simulink model "VIPRExit557StEnCtrl"  (R2018b)
settings: Solver=FixedStepDiscrete  StartTime=0.0  StopTime=10.0  FixedStep=0.01  RelTol=1e-3
undefined symbols (not defined in the file or in its folder): data, KeSMSw4SSecRwLtStLgrstOtwdInwdClosePos1_Val, KeSMSw4SSecRwLtStLgrstUpwdDnwdClosePos1_Val, KeSMSw4SSecRwLtStLgrstUpwdDnwdClosePos2_Val, KeSMSw4SSecRwLtStLgrstUpwdDnwdOpenPos1_Val, PassStBkReclnEn_Clear, PassStBkReclnEn_Set, PassStFwdBkwdEn_Clear, PassStFwdBkwdEn_Set, SecRwRtStBkReclnEn_Clear, SecRwRtStBkReclnEn_Set, SecRwRtStFwdBkwdEn_Clear, SecRwRtStFwdBkwdEn_Set, SecRwRtStLgrstInwdOtwdEn_Clear, SecRwRtStLgrstInwdOtwdEn_Set, SecRwRtStLgrstUpwdDnwdEn_Clear, SecRwRtStLgrstUpwdDnwdEn_Set, ThdRwLtStBkReclnEn_Clear, ThdRwLtStBkReclnEn_Set, ThdRwLtStFwdBkwdEn_Clear, ThdRwLtStFwdBkwdEn_Set, ThdRwRtStBkReclnEn_Clear, ThdRwRtStBkReclnEn_Set, ThdRwRtStFwdBkwdEn_Clear, ThdRwRtStFwdBkwdEn_Set, ZeroREn_Clear, ZeroREn_Set
libraries: simulink x1
settings Model: Creator=sn2xws  LastModifiedBy=sn2xws
settings Model: ModifiedHistory=|
  | 2024.7.4 V3.0.0 557模式流程V1.9
  | 2024.8.21 V3.0.1 增加FirstTrig参数
  | 2024.8.28 V3.0.2 副驾靠背小于目标位置时也要判断完成避免ongoing
  | 2024.9.18 V3.0.3  6s版本不需要动三左座椅，不需要posdone，第三阶段遗漏副驾靠背运动,三排占座不用动三排座椅，第三阶段遗漏三排靠背展开
  | 2024.9.18 V3.0.4 腿托及腿托延伸到位置信号连接错误
  | 2024.9.24 V3.0.5 7s版本三左靠背未到位置就到了下个阶段（进入第二阶段判断is7s改为！is7s），第三阶段未移动三左靠背
  | 2024.10.8 V3.0.6 方向比较常量类型错误
  | 25.9.12 V3.16.0 优化副驾占座逻辑，一旦占座不恢复动作
settings DataIOCC: SaveFormat=StructureWithTime
settings OptimizationCC: DefaultParameterBehavior=Inlined  EnhancedBackFolding=on  PassReuseOutputArgsAs=Individual arguments  ZeroExternalMemoryAtStartup=off  ZeroInternalMemoryAtStartup=off  OptimizeBlockOrder=speed  DifferentSizesBufferReuse=on  OptimizationCustomize=off
settings DebuggingCC: ParameterTunabilityLossMsg=error
settings SFSimCC: MATLABDynamicMemAlloc=off
settings RTWCC: SystemTargetFile=autosar.tlc  GenCodeOnly=on  TemplateMakefile=ert_default_tmf  Description=AUTOSAR  GenerateReport=on  IncludeHyperlinkInReport=on  LaunchReport=on  GenerateTraceInfo=on  GenerateTraceReport=on  GenerateTraceReportSl=on  GenerateTraceReportSf=on  GenerateTraceReportEml=on
settings CodeAppCC: ForceParamTrailComments=on  IgnoreCustomStorageClasses=off  OperatorAnnotations=on  SimulinkDataObjDesc=on  SFDataObjDesc=on  InsertBlockDesc=on
settings STFCustomTargetCC: TargetLangStandard=C99 (ISO)  MultiwordLength=256  ParMdlRefBuildCompliant=on  CompOptLevelCompliant=on  IncludeMdlTerminateFcn=off  CombineOutputUpdateFcns=on  SuppressErrorStatus=on  ERTCustomFileBanners=on  SupportNonFinite=off  SupportComplex=off  SupportContinuousTime=off  SupportNonInlinedSFcns=off  RemoveResetFunc=on  MATLABClassNameForMDSCustomization=Simulink.SoftwareTarget.ERTCustomization  AutosarCompliant=on  UseToolchainInfoCompliant=on  LookupTableObjectStructAxisOrder=2,1,3,4,...  LUTObjectStructOrderEvenSpacing=Size,Table,Breakpoints  SystemTargetFile=autosar.tlc
settings ERTTargetCC: TargetLangStandard=C99 (ISO)  ConcurrentExecutionCompliant=off  IncludeMdlTerminateFcn=off  SuppressErrorStatus=on  SupportNonFinite=off  SupportComplex=off  ModelStepFunctionPrototypeControlCompliant=off  CPPClassGenCompliant=off  AutosarCompliant=on  LookupTableObjectStructAxisOrder=2,1,3,4,...  LUTObjectStructOrderEvenSpacing=Size,Table,Breakpoints  InlinedParameterPlacement=NonHierarchical  ERTCustomFileTemplate=example_file_process.tlc  ERTFilePackagingFormat=Compact

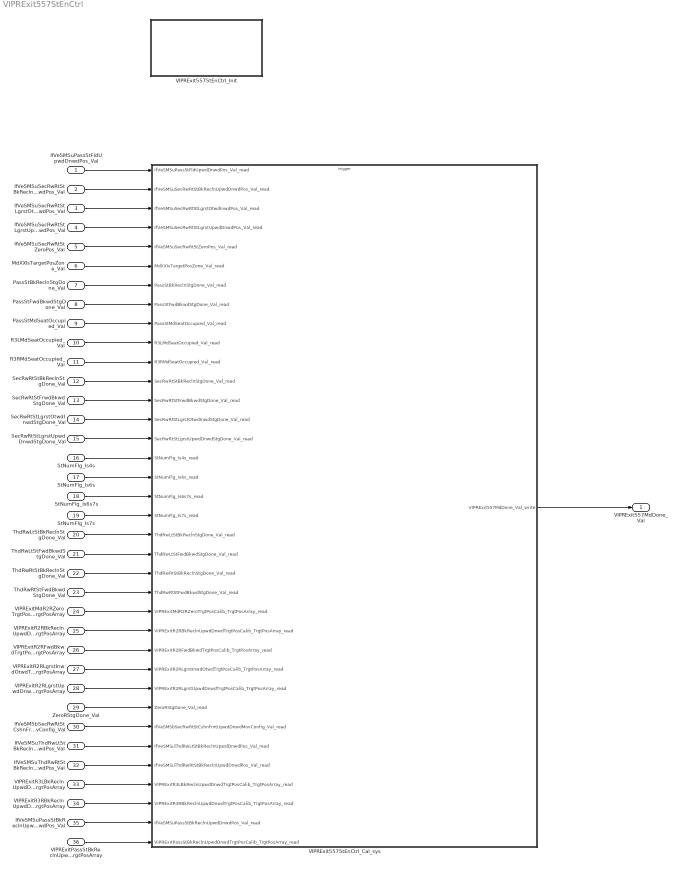
== system VIPRExit557StEnCtrl ==
  IfVeSMSuPassStFldUpwdDnwdPos_Val : Inport  OutDataTypeStr=uint16  PortDimensions=1
  IfVeSMSuSecRwRtStBkReclnUpwdDnwdPos_Val : Inport  Port=2  OutDataTypeStr=uint16  PortDimensions=1
  IfVeSMSuSecRwRtStLgrstOtwdInwdPos_Val : Inport  Port=3  OutDataTypeStr=uint16  PortDimensions=1
  IfVeSMSuSecRwRtStLgrstUpwdDnwdPos_Val : Inport  Port=4  OutDataTypeStr=uint16  PortDimensions=1
  IfVeSMSuSecRwRtStZeroPos_Val : Inport  Port=5  OutDataTypeStr=uint16  PortDimensions=1
  MdXXIsTargetPosZone_Val : Inport  Port=6  OutDataTypeStr=uint32  PortDimensions=1
  PassStBkReclnStgDone_Val : Inport  Port=7  OutDataTypeStr=boolean  PortDimensions=1
  PassStFwdBkwdStgDone_Val : Inport  Port=8  OutDataTypeStr=boolean  PortDimensions=1
  PassStMdSeatOccupied_Val : Inport  Port=9  OutDataTypeStr=boolean  PortDimensions=1
  R3LMdSeatOccupied_Val : Inport  Port=10  OutDataTypeStr=boolean  PortDimensions=1
  R3RMdSeatOccupied_Val : Inport  Port=11  OutDataTypeStr=boolean  PortDimensions=1
  SecRwRtStBkReclnStgDone_Val : Inport  Port=12  OutDataTypeStr=boolean  PortDimensions=1
  SecRwRtStFrwdBkwdStgDone_Val : Inport  Port=13  OutDataTypeStr=boolean  PortDimensions=1
  SecRwRtStLgrstOtwdInwdStgDone_Val : Inport  Port=14  OutDataTypeStr=boolean  PortDimensions=1
  SecRwRtStLgrstUpwdDnwdStgDone_Val : Inport  Port=15  OutDataTypeStr=boolean  PortDimensions=1
  StNumFlg_Is4s : Inport  Port=16  OutDataTypeStr=boolean  PortDimensions=1
  StNumFlg_Is6s : Inport  Port=17  OutDataTypeStr=boolean  PortDimensions=1
  StNumFlg_Is6s7s : Inport  Port=18  OutDataTypeStr=boolean  PortDimensions=1
  StNumFlg_Is7s : Inport  Port=19  OutDataTypeStr=boolean  PortDimensions=1
  ThdRwLtStBkReclnStgDone_Val : Inport  Port=20  OutDataTypeStr=boolean  PortDimensions=1
  ThdRwLtStFwdBkwdStgDone_Val : Inport  Port=21  OutDataTypeStr=boolean  PortDimensions=1
  ThdRwRtStBkReclnStgDone_Val : Inport  Port=22  OutDataTypeStr=boolean  PortDimensions=1
  ThdRwRtStFwdBkwdStgDone_Val : Inport  Port=23  OutDataTypeStr=boolean  PortDimensions=1
  VIPRExitMdR2RZeroTrgtPosCalib_TrgtPosArray : Inport  Description=|  Port=24  OutDataTypeStr=uint16  PortDimensions=3
      | 0:Pos
      | 1:Max
      | 2:Min
  VIPRExitR2RBkReclnUpwdDnwdTrgtPosCalib_TrgtPosArray : Inport  Description=|  Port=25  OutDataTypeStr=uint16  PortDimensions=3
      | 0:Pos
      | 1:Max
      | 2:Min
  VIPRExitR2RFwdBkwdTrgtPosCalib_TrgtPosArray : Inport  Description=|  Port=26  OutDataTypeStr=uint16  PortDimensions=3
      | 0:Pos
      | 1:Max
      | 2:Min
  VIPRExitR2RLgrstInwdOtwdTrgtPosCalib_TrgtPosArray : Inport  Description=|  Port=27  OutDataTypeStr=uint16  PortDimensions=3
      | 0:Pos
      | 1:Max
      | 2:Min
  VIPRExitR2RLgrstUpwdDnwdTrgtPosCalib_TrgtPosArray : Inport  Description=|  Port=28  OutDataTypeStr=uint16  PortDimensions=3
      | 0:Pos
      | 1:Max
      | 2:Min
  ZeroRStgDone_Val : Inport  Port=29  OutDataTypeStr=boolean  PortDimensions=1
  IfVeSMSbSecRwRtStCshnFrntUpwdDnwdMovConfig_Val : Inport  Port=30  OutDataTypeStr=boolean  PortDimensions=1
  IfVeSMSuThdRwLtStBkReclnUpwdDnwdPos_Val : Inport  Port=31  OutDataTypeStr=uint16  PortDimensions=1
  IfVeSMSuThdRwRtStBkReclnUpwdDnwdPos_Val : Inport  Port=32  OutDataTypeStr=uint16  PortDimensions=1
  VIPRExitR3LBkReclnUpwdDnwdTrgtPosCalib_TrgtPosArray : Inport  Description=|  Port=33  OutDataTypeStr=uint16  PortDimensions=3
      | 0:Pos
      | 1:Max
      | 2:Min
  VIPRExitR3RBkReclnUpwdDnwdTrgtPosCalib_TrgtPosArray : Inport  Description=|  Port=34  OutDataTypeStr=uint16  PortDimensions=3
      | 0:Pos
      | 1:Max
      | 2:Min
  IfVeSMSuPassStBkReclnUpwdDnwdPos_Val : Inport  Port=35  OutDataTypeStr=uint16  PortDimensions=1
  VIPRExitPassStBkReclnUpwdDnwdTrgtPosCalib_TrgtPosArray : Inport  Description=|  Port=36  OutDataTypeStr=uint16  PortDimensions=3
      | 0:Pos
      | 1:Max
      | 2:Min
  VIPRExit557StEnCtrl_Cal_sys : Subsystem
  VIPRExit557StEnCtrl_Init : Subsystem
  VIPRExit557MdDone_Val : Outport  OutDataTypeStr=uint8  PortDimensions=1
  wires:
  IfVeSMSuPassStFldUpwdDnwdPos_Val/1 -> VIPRExit557StEnCtrl_Cal_sys/1(IfVeSMSuPassStFldUpwdDnwdPos_Val_read)
  IfVeSMSuSecRwRtStBkReclnUpwdDnwdPos_Val/1 -> VIPRExit557StEnCtrl_Cal_sys/2(IfVeSMSuSecRwRtStBkReclnUpwdDnwdPos_Val_read)
  IfVeSMSuSecRwRtStLgrstOtwdInwdPos_Val/1 -> VIPRExit557StEnCtrl_Cal_sys/3(IfVeSMSuSecRwRtStLgrstOtwdInwdPos_Val_read)
  IfVeSMSuSecRwRtStLgrstUpwdDnwdPos_Val/1 -> VIPRExit557StEnCtrl_Cal_sys/4(IfVeSMSuSecRwRtStLgrstUpwdDnwdPos_Val_read)
  IfVeSMSuSecRwRtStZeroPos_Val/1 -> VIPRExit557StEnCtrl_Cal_sys/5(IfVeSMSuSecRwRtStZeroPos_Val_read)
  MdXXIsTargetPosZone_Val/1 -> VIPRExit557StEnCtrl_Cal_sys/6(MdXXIsTargetPosZone_Val_read)
  PassStBkReclnStgDone_Val/1 -> VIPRExit557StEnCtrl_Cal_sys/7(PassStBkReclnStgDone_Val_read)
  PassStFwdBkwdStgDone_Val/1 -> VIPRExit557StEnCtrl_Cal_sys/8(PassStFwdBkwdStgDone_Val_read)
  PassStMdSeatOccupied_Val/1 -> VIPRExit557StEnCtrl_Cal_sys/9(PassStMdSeatOccupied_Val_read)
  R3LMdSeatOccupied_Val/1 -> VIPRExit557StEnCtrl_Cal_sys/10(R3LMdSeatOccupied_Val_read)
  R3RMdSeatOccupied_Val/1 -> VIPRExit557StEnCtrl_Cal_sys/11(R3RMdSeatOccupied_Val_read)
  SecRwRtStBkReclnStgDone_Val/1 -> VIPRExit557StEnCtrl_Cal_sys/12(SecRwRtStBkReclnStgDone_Val_read)
  SecRwRtStFrwdBkwdStgDone_Val/1 -> VIPRExit557StEnCtrl_Cal_sys/13(SecRwRtStFrwdBkwdStgDone_Val_read)
  SecRwRtStLgrstOtwdInwdStgDone_Val/1 -> VIPRExit557StEnCtrl_Cal_sys/14(SecRwRtStLgrstOtwdInwdStgDone_Val_read)
  SecRwRtStLgrstUpwdDnwdStgDone_Val/1 -> VIPRExit557StEnCtrl_Cal_sys/15(SecRwRtStLgrstUpwdDnwdStgDone_Val_read)
  StNumFlg_Is4s/1 -> VIPRExit557StEnCtrl_Cal_sys/16(StNumFlg_Is4s_read)
  StNumFlg_Is6s/1 -> VIPRExit557StEnCtrl_Cal_sys/17(StNumFlg_Is6s_read)
  StNumFlg_Is6s7s/1 -> VIPRExit557StEnCtrl_Cal_sys/18(StNumFlg_Is6s7s_read)
  StNumFlg_Is7s/1 -> VIPRExit557StEnCtrl_Cal_sys/19(StNumFlg_Is7s_read)
  ThdRwLtStBkReclnStgDone_Val/1 -> VIPRExit557StEnCtrl_Cal_sys/20(ThdRwLtStBkReclnStgDone_Val_read)
  ThdRwLtStFwdBkwdStgDone_Val/1 -> VIPRExit557StEnCtrl_Cal_sys/21(ThdRwLtStFwdBkwdStgDone_Val_read)
  ThdRwRtStBkReclnStgDone_Val/1 -> VIPRExit557StEnCtrl_Cal_sys/22(ThdRwRtStBkReclnStgDone_Val_read)
  ThdRwRtStFwdBkwdStgDone_Val/1 -> VIPRExit557StEnCtrl_Cal_sys/23(ThdRwRtStFwdBkwdStgDone_Val_read)
  VIPRExitMdR2RZeroTrgtPosCalib_TrgtPosArray/1 -> VIPRExit557StEnCtrl_Cal_sys/24(VIPRExitMdR2RZeroTrgtPosCalib_TrgtPosArray_read)
  VIPRExitR2RBkReclnUpwdDnwdTrgtPosCalib_TrgtPosArray/1 -> VIPRExit557StEnCtrl_Cal_sys/25(VIPRExitR2RBkReclnUpwdDnwdTrgtPosCalib_TrgtPosArray_read)
  VIPRExitR2RFwdBkwdTrgtPosCalib_TrgtPosArray/1 -> VIPRExit557StEnCtrl_Cal_sys/26(VIPRExitR2RFwdBkwdTrgtPosCalib_TrgtPosArray_read)
  VIPRExitR2RLgrstInwdOtwdTrgtPosCalib_TrgtPosArray/1 -> VIPRExit557StEnCtrl_Cal_sys/27(VIPRExitR2RLgrstInwdOtwdTrgtPosCalib_TrgtPosArray_read)
  VIPRExitR2RLgrstUpwdDnwdTrgtPosCalib_TrgtPosArray/1 -> VIPRExit557StEnCtrl_Cal_sys/28(VIPRExitR2RLgrstUpwdDnwdTrgtPosCalib_TrgtPosArray_read)
  ZeroRStgDone_Val/1 -> VIPRExit557StEnCtrl_Cal_sys/29(ZeroRStgDone_Val_read)
  VIPRExit557StEnCtrl_Cal_sys/1(VIPRExit557MdDone_Val_write) -> VIPRExit557MdDone_Val/1
  IfVeSMSbSecRwRtStCshnFrntUpwdDnwdMovConfig_Val/1 -> VIPRExit557StEnCtrl_Cal_sys/30(IfVeSMSbSecRwRtStCshnFrntUpwdDnwdMovConfig_Val_read)
  IfVeSMSuThdRwLtStBkReclnUpwdDnwdPos_Val/1 -> VIPRExit557StEnCtrl_Cal_sys/31(IfVeSMSuThdRwLtStBkReclnUpwdDnwdPos_Val_read)
  IfVeSMSuThdRwRtStBkReclnUpwdDnwdPos_Val/1 -> VIPRExit557StEnCtrl_Cal_sys/32(IfVeSMSuThdRwRtStBkReclnUpwdDnwdPos_Val_read)
  VIPRExitR3LBkReclnUpwdDnwdTrgtPosCalib_TrgtPosArray/1 -> VIPRExit557StEnCtrl_Cal_sys/33(VIPRExitR3LBkReclnUpwdDnwdTrgtPosCalib_TrgtPosArray_read)
  VIPRExitR3RBkReclnUpwdDnwdTrgtPosCalib_TrgtPosArray/1 -> VIPRExit557StEnCtrl_Cal_sys/34(VIPRExitR3RBkReclnUpwdDnwdTrgtPosCalib_TrgtPosArray_read)
  IfVeSMSuPassStBkReclnUpwdDnwdPos_Val/1 -> VIPRExit557StEnCtrl_Cal_sys/35(IfVeSMSuPassStBkReclnUpwdDnwdPos_Val_read)
  VIPRExitPassStBkReclnUpwdDnwdTrgtPosCalib_TrgtPosArray/1 -> VIPRExit557StEnCtrl_Cal_sys/36(VIPRExitPassStBkReclnUpwdDnwdTrgtPosCalib_TrgtPosArray_read)

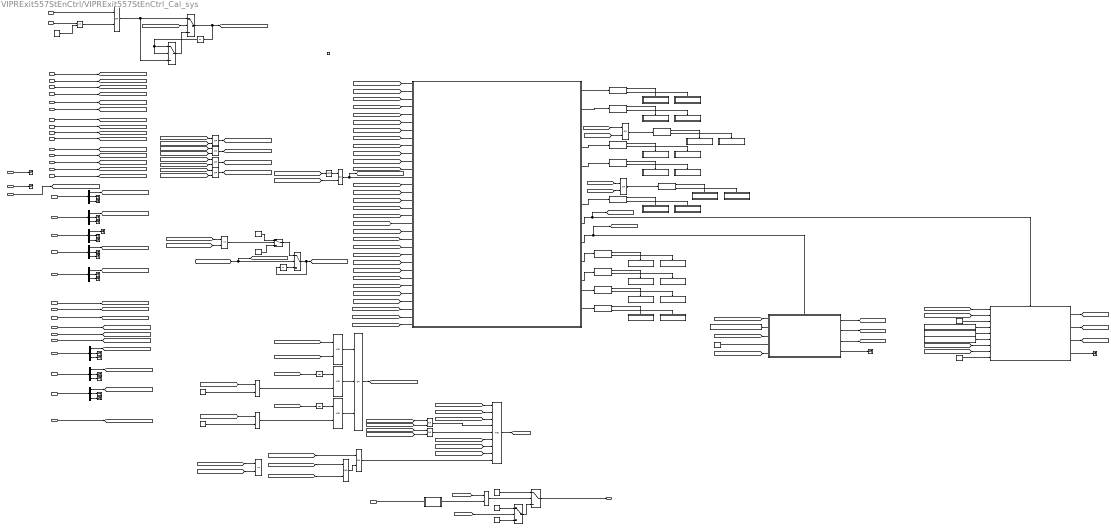
== system VIPRExit557StEnCtrl/VIPRExit557StEnCtrl_Cal_sys ==
  IfVeSMSuPassStFldUpwdDnwdPos_Val_read : Inport
  IfVeSMSuSecRwRtStBkReclnUpwdDnwdPos_Val_read : Inport  Port=2
  IfVeSMSuSecRwRtStLgrstOtwdInwdPos_Val_read : Inport  Port=3
  IfVeSMSuSecRwRtStLgrstUpwdDnwdPos_Val_read : Inport  Port=4
  IfVeSMSuSecRwRtStZeroPos_Val_read : Inport  Port=5
  MdXXIsTargetPosZone_Val_read : Inport  Port=6
  PassStBkReclnStgDone_Val_read : Inport  Port=7
  PassStFwdBkwdStgDone_Val_read : Inport  Port=8
  PassStMdSeatOccupied_Val_read : Inport  Port=9
  R3LMdSeatOccupied_Val_read : Inport  Port=10
  R3RMdSeatOccupied_Val_read : Inport  Port=11
  SecRwRtStBkReclnStgDone_Val_read : Inport  Port=12
  SecRwRtStFrwdBkwdStgDone_Val_read : Inport  Port=13
  SecRwRtStLgrstOtwdInwdStgDone_Val_read : Inport  Port=14
  SecRwRtStLgrstUpwdDnwdStgDone_Val_read : Inport  Port=15
  StNumFlg_Is4s_read : Inport  Port=16
  StNumFlg_Is6s_read : Inport  Port=17
  StNumFlg_Is6s7s_read : Inport  Port=18
  StNumFlg_Is7s_read : Inport  Port=19
  ThdRwLtStBkReclnStgDone_Val_read : Inport  Port=20
  ThdRwLtStFwdBkwdStgDone_Val_read : Inport  Port=21
  ThdRwRtStBkReclnStgDone_Val_read : Inport  Port=22
  ThdRwRtStFwdBkwdStgDone_Val_read : Inport  Port=23
  VIPRExitMdR2RZeroTrgtPosCalib_TrgtPosArray_read : Inport  Port=24
  VIPRExitR2RBkReclnUpwdDnwdTrgtPosCalib_TrgtPosArray_read : Inport  Port=25
  VIPRExitR2RFwdBkwdTrgtPosCalib_TrgtPosArray_read : Inport  Port=26
  VIPRExitR2RLgrstInwdOtwdTrgtPosCalib_TrgtPosArray_read : Inport  Port=27
  VIPRExitR2RLgrstUpwdDnwdTrgtPosCalib_TrgtPosArray_read : Inport  Port=28
  ZeroRStgDone_Val_read : Inport  Port=29
  IfVeSMSbSecRwRtStCshnFrntUpwdDnwdMovConfig_Val_read : Inport  Port=30
  IfVeSMSuThdRwLtStBkReclnUpwdDnwdPos_Val_read : Inport  Port=31
  IfVeSMSuThdRwRtStBkReclnUpwdDnwdPos_Val_read : Inport  Port=32
  VIPRExitR3LBkReclnUpwdDnwdTrgtPosCalib_TrgtPosArray_read : Inport  Port=33
  VIPRExitR3RBkReclnUpwdDnwdTrgtPosCalib_TrgtPosArray_read : Inport  Port=34
  IfVeSMSuPassStBkReclnUpwdDnwdPos_Val_read : Inport  Port=35
  VIPRExitPassStBkReclnUpwdDnwdTrgtPosCalib_TrgtPosArray_read : Inport  Port=36
  function : TriggerPort  TriggerType=function-call  IsSimulinkFunction=on  FunctionName=VIPRExit557StEnCtrl_Cal  VariantControl=(inherit)
  32BitSelector : Subsystem  mask(32 Bit Selector){BitNum=27}
      mask prompts: BitNum "Select Bit Number"
      mask help: Allows selection of a particular bit (0-31) out of a packed word up to 32 bits long. Output will be true if the bit number selected via the mask parameter is equal to one.
      mask TypeOptions BitNum: 0 | 1 | 2 | 3 | 4 | 5 | 6 | 7 | 8 | 9 | 10 | 11 | 12 | 13 | 14 | 15 | 16 | 17 | 18 | 19 | 20 | 21 | 22 | 23 | 24 | 25 | 26 | 27 | 28 | 29 | 30 | 31
      mask Display:
      | text(0.5, 0.8,'BIT','horizontalAlignment','center')
      | text(0.5, 0.5,'SELECTOR','horizontalAlignment','center')
      | text(0.5, 0.2,['-- Bit ',char(get_param(gcb,'BitNum')),' --'],'horizontalAlignment','center')
  Chart : Stateflow chart  TreatAsAtomicUnit=on
  Constant : Constant  OutDataTypeStr=uint8
  Constant1 : Constant  Value=2  OutDataTypeStr=uint8
  Constant10 : Constant  OutDataTypeStr=uint8
  Constant11 : Constant  Value=0  OutDataTypeStr=uint16
  Constant2 : Constant  Value=0  OutDataTypeStr=uint8
  Constant3 : Constant  OutDataTypeStr=boolean
  Constant4 : Constant  OutDataTypeStr=boolean
  Constant5 : Constant  Value=0  OutDataTypeStr=uint16
  Constant7 : Constant  OutDataTypeStr=uint8
  Constant8 : Constant  Value=2  OutDataTypeStr=uint8
  Constant9 : Constant  Value=2  OutDataTypeStr=uint8
  Demux{,1..7} (8 alike) : Demux  Outputs=3
  If Action Subsystem1 : Subsystem  TreatAsAtomicUnit=on
  If Action Subsystem10 : Subsystem  TreatAsAtomicUnit=on
  If Action Subsystem11 : Subsystem  TreatAsAtomicUnit=on
  If Action Subsystem12 : Subsystem  TreatAsAtomicUnit=on
  If Action Subsystem13 : Subsystem  TreatAsAtomicUnit=on
  If Action Subsystem14 : Subsystem  TreatAsAtomicUnit=on
  If Action Subsystem15 : Subsystem  TreatAsAtomicUnit=on
  If Action Subsystem16 : Subsystem  TreatAsAtomicUnit=on
  If Action Subsystem17 : Subsystem  TreatAsAtomicUnit=on
  If Action Subsystem18 : Subsystem  TreatAsAtomicUnit=on
  If Action Subsystem19 : Subsystem  TreatAsAtomicUnit=on
  If Action Subsystem2 : Subsystem  TreatAsAtomicUnit=on
  If Action Subsystem20 : Subsystem  TreatAsAtomicUnit=on
  If Action Subsystem21 : Subsystem  TreatAsAtomicUnit=on
  If Action Subsystem22 : Subsystem  TreatAsAtomicUnit=on
  If Action Subsystem3 : Subsystem  TreatAsAtomicUnit=on
  If Action Subsystem4 : Subsystem  TreatAsAtomicUnit=on
  If Action Subsystem5 : Subsystem  TreatAsAtomicUnit=on
  If Action Subsystem6 : Subsystem  TreatAsAtomicUnit=on
  If Action Subsystem7 : Subsystem  TreatAsAtomicUnit=on
  If Action Subsystem8 : Subsystem  TreatAsAtomicUnit=on
  If Action Subsystem9 : Subsystem  TreatAsAtomicUnit=on
  If{1..11} (11 alike) : If  IfExpression=u1
  LgrstClose : Subsystem
  LgrstOpen : Subsystem
  Logical Operator : Logic  Operator=NOT  AllPortsSameDT=off  OutDataTypeStr=boolean
  Logical Operator{1,3..4,12..19} (11 alike) : Logic  Operator=OR  AllPortsSameDT=off  OutDataTypeStr=boolean
  Logical Operator10 : Logic  Inputs=9  AllPortsSameDT=off  OutDataTypeStr=boolean
  Logical Operator{2,6..7,9,11} (5 alike) : Logic  AllPortsSameDT=off  OutDataTypeStr=boolean
  Logical Operator5 : Logic  Operator=OR  Inputs=3  AllPortsSameDT=off  OutDataTypeStr=boolean
  PA_KeSMSw4SSecRwLtStLgrstOtwdInwdClosePos1_Val : Constant  Value=KeSMSw4SSecRwLtStLgrstOtwdInwdClosePos1_Val
  PA_KeSMSw4SSecRwLtStLgrstUpwdDnwdClosePos1_Val : Constant  Value=KeSMSw4SSecRwLtStLgrstUpwdDnwdClosePos1_Val
  PA_KeSMSw4SSecRwLtStLgrstUpwdDnwdClosePos2_Val : Constant  Value=KeSMSw4SSecRwLtStLgrstUpwdDnwdClosePos2_Val
  PA_KeSMSw4SSecRwLtStLgrstUpwdDnwdOpenPos1_Val1 : Constant  Value=KeSMSw4SSecRwLtStLgrstUpwdDnwdOpenPos1_Val
  Relational Operator : RelationalOperator  OutDataTypeStr=boolean  RndMeth=Simplest
  Relational Operator1 : RelationalOperator  Operator===  OutDataTypeStr=boolean  RndMeth=Simplest
  Relational Operator2 : RelationalOperator  Operator=<=  OutDataTypeStr=boolean  RndMeth=Simplest
  Relational Operator3 : RelationalOperator  Operator===  OutDataTypeStr=boolean  RndMeth=Simplest
  Relational Operator4 : RelationalOperator  Operator=<=  OutDataTypeStr=boolean  RndMeth=Simplest
  Switch{,1..5} (6 alike) : Switch  Criteria=u2 > Threshold
  Terminator{,1..10,12..21} (21 alike) : Terminator
  Unit Delay{,1,3..4} (4 alike) : UnitDelay  SampleTime=-1
  FirstTrig : ArgIn  OutDataTypeStr=boolean  ArgumentName=FirstTrig
  VIPRExit557MdDone_Val_write : Outport
      settings: EnsureOutportIsVirtual=on
  wires:
  Switch/1 -> VIPRExit557MdDone_Val_write/1
  ZeroRStgDone_Val_read/1 -> [ZeroRStgDone]
  PassStFwdBkwdStgDone_Val_read/1 -> [PassStFwdBkwdStgDone]
  IfVeSMSuSecRwRtStZeroPos_Val_read/1 -> [IfVeSMSuSecRwRtStZeroPos]
  SecRwRtStFrwdBkwdStgDone_Val_read/1 -> [SecRwRtStFrwdBkwdStgDone]
  ThdRwLtStBkReclnStgDone_Val_read/1 -> [ThdRwLtStBkReclnStgDone]
  IfVeSMSuSecRwRtStLgrstUpwdDnwdPos_Val_read/1 -> [IfVeSMSuSecRwRtStLgrstUpwdDnwdPos]
  IfVeSMSuSecRwRtStLgrstOtwdInwdPos_Val_read/1 -> [IfVeSMSuSecRwRtStLgrstOtwdInwdPos]
  ThdRwLtStFwdBkwdStgDone_Val_read/1 -> [ThdRwLtStFwdBkwdStgDone]
  SecRwRtStBkReclnStgDone_Val_read/1 -> [SecRwRtStBkReclnStgDone]
  IfVeSMSuSecRwRtStBkReclnUpwdDnwdPos_Val_read/1 -> [IfVeSMSuSecRwRtStBkReclnUpwdDnwdPos]
  PassStBkReclnStgDone_Val_read/1 -> [PassStBkReclnStgDone]
  ThdRwRtStBkReclnStgDone_Val_read/1 -> [ThdRwRtStBkReclnStgDone]
  ThdRwRtStFwdBkwdStgDone_Val_read/1 -> [ThdRwRtStFwdBkwdStgDone]
  VIPRExitR2RFwdBkwdTrgtPosCalib_TrgtPosArray_read/1 -> Demux1/1
  Demux1/3 -> Terminator3/1
  Demux/2 -> Terminator/1
  Demux3/2 -> Terminator6/1
  Demux2/2 -> Terminator4/1
  Demux1/1 -> Terminator15/1
  Demux4/2 -> Terminator8/1
  Demux/3 -> Terminator1/1
  VIPRExitMdR2RZeroTrgtPosCalib_TrgtPosArray_read/1 -> Demux4/1
  VIPRExitR2RLgrstUpwdDnwdTrgtPosCalib_TrgtPosArray_read/1 -> Demux3/1
  Demux3/1 -> [VIPRR2RLgrstUpwdDnwdTrgtPos]
  Demux1/2 -> Terminator2/1
  Demux2/1 -> [VIPRR2RLgrstInwdOtwdTrgtPos]
  Demux3/3 -> Terminator7/1
  VIPRExitR2RLgrstInwdOtwdTrgtPosCalib_TrgtPosArray_read/1 -> Demux2/1
  Demux2/3 -> Terminator5/1
  Demux/1 -> [VIPRR2RBkReclnUpwdDnwdTrgtPos]
  Demux4/1 -> [VIPRMdR2RZeroTrgtPos]
  VIPRExitR2RBkReclnUpwdDnwdTrgtPosCalib_TrgtPosArray_read/1 -> Demux/1
  Demux4/3 -> Terminator9/1
  StNumFlg_Is4s_read/1 -> Terminator10/1
  StNumFlg_Is6s_read/1 -> [is6s]
  StNumFlg_Is6s7s_read/1 -> Terminator12/1
  R3LMdSeatOccupied_Val_read/1 -> [R3LMdSeatOccupied]
  R3RMdSeatOccupied_Val_read/1 -> [R3RMdSeatOccupied]
  StNumFlg_Is7s_read/1 -> [StNumFlg_Is7s]
  MdXXIsTargetPosZone_Val_read/1 -> 32BitSelector/1(x)
  [AllDone] -> Logical Operator9/1
  Constant1/1 -> Switch1/1
  [AllDone] -> Switch1/2
  Switch1/1 -> Switch/3
  Constant/1 -> Switch/1
  Logical Operator9/1 -> Switch/2
  32BitSelector/1(y) -> Logical Operator9/2
  Constant2/1 -> Switch1/3
  PA_KeSMSw4SSecRwLtStLgrstUpwdDnwdOpenPos1_Val1/1 -> LgrstOpen/2(LgrstUpwdDnwdOpenPos1)
  PA_KeSMSw4SSecRwLtStLgrstUpwdDnwdClosePos2_Val/1 -> LgrstClose/5(LgrstUpwdDnwdClosePos2)
  Constant5/1 -> LgrstClose/3(FtupwdDnwdPos)
  Constant4/1 -> LgrstClose/9(FtrstStgDone)
  [IfVeSMSuSecRwRtStLgrstOtwdInwdPos] -> LgrstClose/2(LgrstInwdOtwdPos)
  Logical Operator3/1 -> If4/1
  Chart/9(LgrstOpnEn) -> [LgrstOpnEn], LgrstOpen/Enable
  If1/2 -> If Action Subsystem1/Action
  Chart/5(ThdRwLtStFwdBkwdEn) -> If3/1
  LgrstOpen/4(FtrstEn) -> Terminator14/1
  PA_KeSMSw4SSecRwLtStLgrstOtwdInwdClosePos1_Val/1 -> LgrstClose/6(LgrstInwdOtWdPos1)
  Chart/8(LgrstClsEn) -> LgrstClose/Enable, [LgrstClsEn]
  [LgrstUpwdEn3] -> Logical Operator3/2
  Chart/2(SecRwLtStFrwdBkwdEn) -> If1/1
  Logical Operator4/1 -> If5/1
  Chart/1(SecRwLtStBkReclnEn) -> If8/1
  LgrstOpen/1(Failflg) -> [FailflgOpn]
  If1/1 -> If Action Subsystem2/Action
  If5/1 -> If Action Subsystem10/Action
  [LgrstInwdOtwdEn3] -> Logical Operator4/2
  If3/2 -> If Action Subsystem5/Action
  LgrstOpen/2(LgrstInwdOtwdEn) -> [LgrstInwdOtwdEn2]
  [IfVeSMSuSecRwRtStLgrstUpwdDnwdPos] -> LgrstClose/1(LgrstUpwdDnwdPos)
  If6/1 -> If Action Subsystem13/Action
  [LgrstInwdOtwdEn2] -> Logical Operator4/1
  If8/1 -> If Action Subsystem14/Action
  Constant3/1 -> LgrstOpen/4(FtrstStgDone)
  Chart/4(ThdRwLtStBkReclnEn) -> If2/1
  If2/1 -> If Action Subsystem4/Action
  If4/1 -> If Action Subsystem8/Action
  If8/2 -> If Action Subsystem11/Action
  [SecRwRtStLgrstUpwdDnwdStgDone] -> LgrstOpen/3(LgrstUpwdStgDone)
  PA_KeSMSw4SSecRwLtStLgrstUpwdDnwdClosePos1_Val/1 -> LgrstClose/4(LgrstUpwdDnwdClosePos1)
  If2/2 -> If Action Subsystem3/Action
  If5/2 -> If Action Subsystem9/Action
  If4/2 -> If Action Subsystem7/Action
  [LgrstUpwdEn2] -> Logical Operator3/1
  [SecRwRtStLgrstOtwdInwdStgDone] -> LgrstOpen/5(LgrstInwdStgDone)
  LgrstClose/2(LgrstInwdOtwdEn) -> [LgrstInwdOtwdEn3]
  If3/1 -> If Action Subsystem6/Action
  LgrstClose/4(FtrstEn) -> Terminator13/1
  [IfVeSMSuSecRwRtStLgrstUpwdDnwdPos] -> LgrstOpen/1(LgrstUpwdDnwdPos)
  LgrstOpen/3(LgrstUpwdDnwdEn) -> [LgrstUpwdEn2]
  Chart/7(ZeroLEn) -> If6/1
  [SecRwRtStLgrstUpwdDnwdStgDone] -> LgrstClose/8(LgrstUpwdStgDone)
  LgrstClose/3(LgrstUpwdDnwdEn) -> [LgrstUpwdEn3]
  [SecRwRtStLgrstOtwdInwdStgDone] -> LgrstClose/7(LgrstInwdStgDone)
  LgrstClose/1(Failflg) -> [FailflgCls]
  If6/2 -> If Action Subsystem12/Action
  [LgrstMoveDirection] -> Chart/19(LgrstMoveDirection)
  [SecRwRtStFrwdBkwdStgDone] -> Chart/5(SecRwLtStFrwdBkwdStgDone)
  [ThdRwLtStFwdBkwdStgDoneModify] -> Chart/9(ThdRwLtStFwdBkwdStgDone)
  [IfVeSMSuSecRwRtStLgrstOtwdInwdPos] -> Chart/2(IfVeSMSuSecRwLtStLgrstOtwdInwdPos)
  [IfVeSMSuThdRwLtStBkReclnUpwdDnwdPos] -> Chart/18(IfVeSMSuThdRwLtStBkReclnUpwdDnwdPos)
  [IfVeSMSuSecRwRtStLgrstUpwdDnwdPos] -> Relational Operator/1
  Relational Operator/1 -> Switch2/2
  [LgrstStgDone] -> Chart/17(LgrstStgDone)
  [VIPRR2RLgrstUpwdDnwdTrgtPos] -> Relational Operator/2
  [IfVeSMSuSecRwRtStZeroPos] -> Chart/14(IfVeSMSuSecRwLtStZeroPos)
  [R3LMdSeatOccupied] -> Chart/16(R3LMdSeatOccupied)
  [IfVeSMSbSecRwRtStCshnFrntUpwdDnwdMovConfig] -> Logical Operator/1
  [ZeroRStgDone] -> Logical Operator1/2
  Constant8/1 -> Switch2/3
  [VIPRR2RLgrstInwdOtwdTrgtPos] -> Chart/11(VIPLR2LLgrstInwdOtwdTrgtPos)
  [ThdRwLtStBkReclnStgDoneModify] -> Chart/8(ThdRwLtStBkReclnStgDone)
  [VIPRR2RLgrstUpwdDnwdTrgtPos] -> Chart/12(VIPLR2LLgrstUpwdDnwdTrgtPos)
  [SecRwRtStLgrstUpwdDnwdStgDone] -> Chart/7(SecRwLtStLgrstUpwdDnwdStgDone)
  [IfVeSMSuSecRwRtStBkReclnUpwdDnwdPos] -> Chart/1(IfVeSMSuSecRwLtStBkReclnUpwdDnwdPos)
  Constant7/1 -> Switch2/1
  Logical Operator1/1 -> [ZeroRStgDoneModify], Chart/13(ZeroLStgDone)
  [SecRwRtStBkReclnStgDone] -> Chart/4(SecRwLtStBkReclnStgDone)
  Logical Operator/1 -> Logical Operator1/1
  [SecRwRtStLgrstOtwdInwdStgDone] -> Chart/6(SecRwLtStLgrstOtwdInwdStgDone)
  [VIPRMdR2RZeroTrgtPos] -> Chart/15(VIPLMdR2LZeroTrgtPos)
  [IfVeSMSuSecRwRtStLgrstUpwdDnwdPos] -> Chart/3(IfVeSMSuSecRwLtStLgrstUpwdDnwdPos)
  [VIPRR2RBkReclnUpwdDnwdTrgtPos] -> Chart/10(VIPLR2LBkReclnUpwdDnwdTrgtPos)
  IfVeSMSuPassStFldUpwdDnwdPos_Val_read/1 -> Relational Operator2/1
  IfVeSMSbSecRwRtStCshnFrntUpwdDnwdMovConfig_Val_read/1 -> [IfVeSMSbSecRwRtStCshnFrntUpwdDnwdMovConfig]
  IfVeSMSuThdRwLtStBkReclnUpwdDnwdPos_Val_read/1 -> [IfVeSMSuThdRwLtStBkReclnUpwdDnwdPos]
  IfVeSMSuThdRwRtStBkReclnUpwdDnwdPos_Val_read/1 -> [IfVeSMSuThdRwRtStBkReclnUpwdDnwdPos]
  [IfVeSMSuThdRwRtStBkReclnUpwdDnwdPos] -> Chart/20(IfVeSMSuThdRwRtStBkReclnUpwdDnwdPos)
  [NotMovPassStFlg] -> Chart/21(NotMovPassStFlg)
  [R3RMdSeatOccupied] -> Chart/22(R3RMdSeatOccupied)
  [StNumFlg_Is7s] -> Chart/23(StNumFlg_Is7s)
  [PassStBkReclnStgDone] -> Chart/24(PassStBkReclnStgDone)
  [PassStFwdBkwdStgDone] -> Chart/25(PassStFwdBkwdStgDone)
  [ThdRwRtStBkReclnStgDoneModify] -> Chart/26(ThdRwRtStBkReclnStgDone)
  [ThdRwRtStFwdBkwdStgDoneModify] -> Chart/27(ThdRwRtStFwdBkwdStgDone)
  [VIPRExitR3LBkReclnUpwdDnwdTrgtPos] -> Chart/28(VIPRExitR3LBkReclnUpwdDnwdTrgtPos)
  Demux5/3 -> Terminator17/1
  Demux5/1 -> [VIPRExitR3LBkReclnUpwdDnwdTrgtPos]
  VIPRExitR3LBkReclnUpwdDnwdTrgtPosCalib_TrgtPosArray_read/1 -> Demux5/1
  Demux5/2 -> Terminator16/1
  Demux6/2 -> Terminator18/1
  VIPRExitR3RBkReclnUpwdDnwdTrgtPosCalib_TrgtPosArray_read/1 -> Demux6/1
  Demux6/1 -> [VIPRExitR3RBkReclnUpwdDnwdTrgtPos]
  Demux6/3 -> Terminator19/1
  [VIPRExitR3RBkReclnUpwdDnwdTrgtPos] -> Chart/29(VIPRExitR3RBkReclnUpwdDnwdTrgtPos)
  Logical Operator5/1 -> [LgrstStgDone]
  [LgrstStgDone] -> Logical Operator10/1
  [SecRwRtStLgrstOtwdInwdStgDone] -> Logical Operator2/2
  [SecRwRtStLgrstUpwdDnwdStgDone] -> Logical Operator2/1
  Logical Operator6/1 -> Logical Operator5/2
  Logical Operator10/1 -> [AllDone]
  [SecRwRtStBkReclnStgDone] -> Logical Operator10/2
  [SecRwRtStFrwdBkwdStgDone] -> Logical Operator10/3
  Logical Operator7/1 -> Logical Operator5/3
  Unit Delay4/1 -> Logical Operator7/1
  [FailflgCls] -> Unit Delay4/1
  [FailflgOpn] -> Unit Delay3/1
  [ZeroRStgDoneModify] -> Logical Operator10/6
  Unit Delay3/1 -> Logical Operator6/1
  Logical Operator2/1 -> Logical Operator5/1
  [ThdRwRtStBkReclnStgDoneModify] -> Logical Operator10/7
  [ThdRwRtStFwdBkwdStgDoneModify] -> Logical Operator10/8
  [NotMovPassStFlg] -> Logical Operator13/1
  [PassStFwdBkwdStgDone] -> Logical Operator11/2
  Logical Operator11/1 -> Logical Operator13/2
  Logical Operator13/1 -> Logical Operator10/9
  If7/2 -> If Action Subsystem15/Action
  If7/1 -> If Action Subsystem16/Action
  Chart/10(ThdRwRtStBkReclnEn) -> If7/1
  Chart/11(ThdRwRtStFwdBkwdEn) -> If9/1
  If9/1 -> If Action Subsystem18/Action
  If9/2 -> If Action Subsystem17/Action
  If10/2 -> If Action Subsystem19/Action
  If10/1 -> If Action Subsystem20/Action
  Chart/12(PassStFwdBkwdEn) -> If10/1
  Chart/13(PassStBkReclnEn) -> If11/1
  If11/1 -> If Action Subsystem22/Action
  If11/2 -> If Action Subsystem21/Action
  Constant11/1 -> Relational Operator2/2
  IfVeSMSuPassStBkReclnUpwdDnwdPos_Val_read/1 -> [IfVeSMSuPassStBkReclnUpwdDnwdPos]
  Demux7/3 -> Terminator21/1
  Demux7/1 -> [VIPRExitPassStBkReclnUpwdDnwdTrgtPos]
  VIPRExitPassStBkReclnUpwdDnwdTrgtPosCalib_TrgtPosArray_read/1 -> Demux7/1
  Demux7/2 -> Terminator20/1
  [VIPRExitPassStBkReclnUpwdDnwdTrgtPos] -> Chart/30(VIPRExitPassStBkReclnUpwdDnwdTrgtPos)
  [IfVeSMSuPassStBkReclnUpwdDnwdPos] -> Chart/31(IfVeSMSuPassStBkReclnUpwdDnwdPos)
  [StNumFlg_Is7s] -> Chart/32(Is7s)
  [LgrstMoveDirection] -> Relational Operator1/1
  Relational Operator1/1 -> Logical Operator6/2
  Constant9/1 -> Relational Operator1/2
  Relational Operator3/1 -> Logical Operator7/2
  Constant10/1 -> Relational Operator3/2
  [LgrstMoveDirection] -> Relational Operator3/1
  FirstTrig/1 -> [FirstTrig], Switch3/2
  Switch2/1 -> Switch3/1
  Switch3/1 -> Unit Delay/1, [LgrstMoveDirection]
  Unit Delay/1 -> Switch3/3
  [IfVeSMSuPassStBkReclnUpwdDnwdPos] -> Relational Operator4/1
  [VIPRExitPassStBkReclnUpwdDnwdTrgtPos] -> Relational Operator4/2
  [PassStBkReclnStgDone] -> Logical Operator11/1
  [ThdRwLtStBkReclnStgDoneModify] -> Logical Operator12/1
  Logical Operator12/1 -> Logical Operator10/4
  Logical Operator15/1 -> Logical Operator10/5
  [ThdRwLtStFwdBkwdStgDoneModify] -> Logical Operator15/1
  [is6s] -> Logical Operator12/2
  [is6s] -> Logical Operator15/2
  [R3LMdSeatOccupied] -> Logical Operator16/1
  [ThdRwLtStBkReclnStgDone] -> Logical Operator16/2
  [R3LMdSeatOccupied] -> Logical Operator17/1
  [ThdRwLtStFwdBkwdStgDone] -> Logical Operator17/2
  [R3RMdSeatOccupied] -> Logical Operator18/1
  [ThdRwRtStBkReclnStgDone] -> Logical Operator18/2
  [R3RMdSeatOccupied] -> Logical Operator19/1
  [ThdRwRtStFwdBkwdStgDone] -> Logical Operator19/2
  Logical Operator16/1 -> [ThdRwLtStBkReclnStgDoneModify]
  Logical Operator17/1 -> [ThdRwLtStFwdBkwdStgDoneModify]
  Logical Operator18/1 -> [ThdRwRtStBkReclnStgDoneModify]
  Logical Operator19/1 -> [ThdRwRtStFwdBkwdStgDoneModify]
  SecRwRtStLgrstOtwdInwdStgDone_Val_read/1 -> [SecRwRtStLgrstOtwdInwdStgDone]
  SecRwRtStLgrstUpwdDnwdStgDone_Val_read/1 -> [SecRwRtStLgrstUpwdDnwdStgDone]
  PassStMdSeatOccupied_Val_read/1 -> Logical Operator14/1
  Relational Operator2/1 -> Logical Operator14/2
  [FirstTrig] -> Switch4/2
  Logical Operator14/1 -> Switch5/3, Switch4/1
  Switch4/1 -> Unit Delay1/1, [NotMovPassStFlg]
  Unit Delay1/1 -> Switch5/1, Switch5/2
  Switch5/1 -> Switch4/3

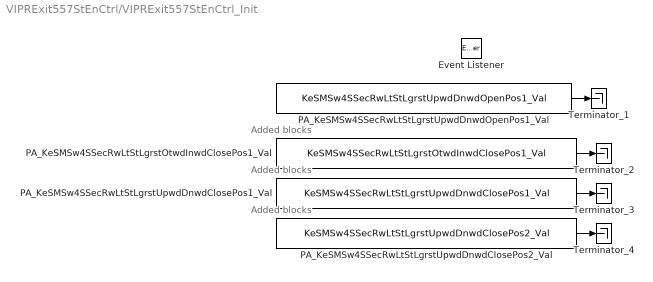
== system VIPRExit557StEnCtrl/VIPRExit557StEnCtrl_Init ==
  note: Added blocks
  note: Added blocks
  note: Added blocks
  Event Listener : EventListener  EventName=reset
  PA_KeSMSw4SSecRwLtStLgrstOtwdInwdClosePos1_Val : Constant  Value=KeSMSw4SSecRwLtStLgrstOtwdInwdClosePos1_Val
  PA_KeSMSw4SSecRwLtStLgrstUpwdDnwdClosePos1_Val : Constant  Value=KeSMSw4SSecRwLtStLgrstUpwdDnwdClosePos1_Val
  PA_KeSMSw4SSecRwLtStLgrstUpwdDnwdClosePos2_Val : Constant  Value=KeSMSw4SSecRwLtStLgrstUpwdDnwdClosePos2_Val
  PA_KeSMSw4SSecRwLtStLgrstUpwdDnwdOpenPos1_Val : Constant  Value=KeSMSw4SSecRwLtStLgrstUpwdDnwdOpenPos1_Val
  Terminator_{1..4} (4 alike) : Terminator
  wires:
  PA_KeSMSw4SSecRwLtStLgrstUpwdDnwdOpenPos1_Val/1 -> Terminator_1/1
  PA_KeSMSw4SSecRwLtStLgrstOtwdInwdClosePos1_Val/1 -> Terminator_2/1
  PA_KeSMSw4SSecRwLtStLgrstUpwdDnwdClosePos1_Val/1 -> Terminator_3/1
  PA_KeSMSw4SSecRwLtStLgrstUpwdDnwdClosePos2_Val/1 -> Terminator_4/1

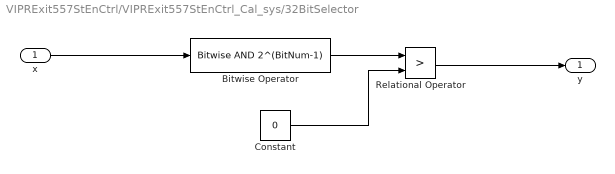
== system VIPRExit557StEnCtrl/VIPRExit557StEnCtrl_Cal_sys/32BitSelector ==
  x : Inport
  Bitwise Operator : simulink/Logic and Bit Operations/Bitwise Operator  logicop=AND  UseBitMask=on  BitMask=2^(BitNum-1)  BitMaskRealWorld=Stored Integer
  Constant : Constant  Value=0  OutDataTypeStr=uint32
  Relational Operator : RelationalOperator  Operator=>  OutDataTypeStr=boolean  RndMeth=Simplest
  y : Outport
  wires:
  Relational Operator/1 -> y/1
  Constant/1 -> Relational Operator/2
  x/1 -> Bitwise Operator/1
  Bitwise Operator/1 -> Relational Operator/1

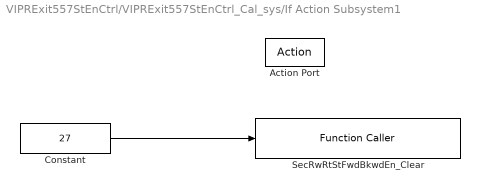
== system VIPRExit557StEnCtrl/VIPRExit557StEnCtrl_Cal_sys/If Action Subsystem1 ==
  Action Port : ActionPort  ActionType=else
  Constant : Constant  Value=27  OutDataTypeStr=uint8
  SecRwRtStFwdBkwdEn_Clear : FunctionCaller  FunctionPrototype=SecRwRtStFwdBkwdEn_Clear(data)  InputArgumentSpecifications=uint8(1)
  wires:
  Constant/1 -> SecRwRtStFwdBkwdEn_Clear/1

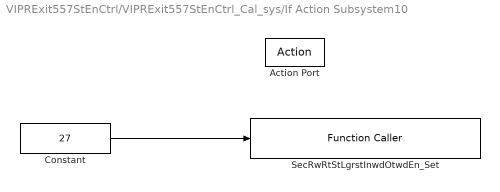
== system VIPRExit557StEnCtrl/VIPRExit557StEnCtrl_Cal_sys/If Action Subsystem10 ==
  Action Port : ActionPort  ActionType=then
  Constant : Constant  Value=27  OutDataTypeStr=uint8
  SecRwRtStLgrstInwdOtwdEn_Set : FunctionCaller  FunctionPrototype=SecRwRtStLgrstInwdOtwdEn_Set(data)  InputArgumentSpecifications=uint8(1)
  wires:
  Constant/1 -> SecRwRtStLgrstInwdOtwdEn_Set/1

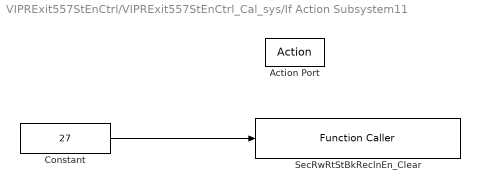
== system VIPRExit557StEnCtrl/VIPRExit557StEnCtrl_Cal_sys/If Action Subsystem11 ==
  Action Port : ActionPort  ActionType=else
  Constant : Constant  Value=27  OutDataTypeStr=uint8
  SecRwRtStBkReclnEn_Clear : FunctionCaller  FunctionPrototype=SecRwRtStBkReclnEn_Clear(data)  InputArgumentSpecifications=uint8(1)
  wires:
  Constant/1 -> SecRwRtStBkReclnEn_Clear/1

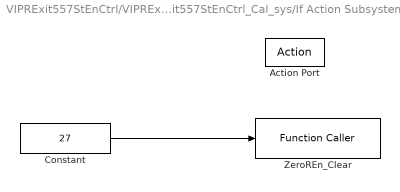
== system VIPRExit557StEnCtrl/VIPRExit557StEnCtrl_Cal_sys/If Action Subsystem12 ==
  Action Port : ActionPort  ActionType=else
  Constant : Constant  Value=27  OutDataTypeStr=uint8
  ZeroREn_Clear : FunctionCaller  FunctionPrototype=ZeroREn_Clear(data)  InputArgumentSpecifications=uint8(1)
  wires:
  Constant/1 -> ZeroREn_Clear/1

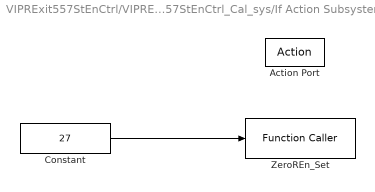
== system VIPRExit557StEnCtrl/VIPRExit557StEnCtrl_Cal_sys/If Action Subsystem13 ==
  Action Port : ActionPort  ActionType=then
  Constant : Constant  Value=27  OutDataTypeStr=uint8
  ZeroREn_Set : FunctionCaller  FunctionPrototype=ZeroREn_Set(data)  InputArgumentSpecifications=uint8(1)
  wires:
  Constant/1 -> ZeroREn_Set/1

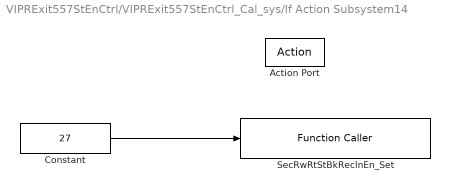
== system VIPRExit557StEnCtrl/VIPRExit557StEnCtrl_Cal_sys/If Action Subsystem14 ==
  Action Port : ActionPort  ActionType=then
  Constant : Constant  Value=27  OutDataTypeStr=uint8
  SecRwRtStBkReclnEn_Set : FunctionCaller  FunctionPrototype=SecRwRtStBkReclnEn_Set(data)  InputArgumentSpecifications=uint8(1)
  wires:
  Constant/1 -> SecRwRtStBkReclnEn_Set/1

== system VIPRExit557StEnCtrl/VIPRExit557StEnCtrl_Cal_sys/If Action Subsystem15 ==
  Action Port : ActionPort  ActionType=else
  Constant : Constant  Value=27  OutDataTypeStr=uint8
  ThdRwRtStBkReclnEn_Clear : FunctionCaller  FunctionPrototype=ThdRwRtStBkReclnEn_Clear(data)  InputArgumentSpecifications=uint8(1)
  wires:
  Constant/1 -> ThdRwRtStBkReclnEn_Clear/1

== system VIPRExit557StEnCtrl/VIPRExit557StEnCtrl_Cal_sys/If Action Subsystem16 ==
  Action Port : ActionPort  ActionType=then
  Constant : Constant  Value=27  OutDataTypeStr=uint8
  ThdRwRtStBkReclnEn_Set : FunctionCaller  FunctionPrototype=ThdRwRtStBkReclnEn_Set(data)  InputArgumentSpecifications=uint8(1)
  wires:
  Constant/1 -> ThdRwRtStBkReclnEn_Set/1

== system VIPRExit557StEnCtrl/VIPRExit557StEnCtrl_Cal_sys/If Action Subsystem17 ==
  Action Port : ActionPort  ActionType=else
  Constant : Constant  Value=27  OutDataTypeStr=uint8
  ThdRwRtStFwdBkwdEn_Clear : FunctionCaller  FunctionPrototype=ThdRwRtStFwdBkwdEn_Clear(data)  InputArgumentSpecifications=uint8(1)
  wires:
  Constant/1 -> ThdRwRtStFwdBkwdEn_Clear/1

== system VIPRExit557StEnCtrl/VIPRExit557StEnCtrl_Cal_sys/If Action Subsystem18 ==
  Action Port : ActionPort  ActionType=then
  Constant : Constant  Value=27  OutDataTypeStr=uint8
  ThdRwRtStFwdBkwdEn_Set : FunctionCaller  FunctionPrototype=ThdRwRtStFwdBkwdEn_Set(data)  InputArgumentSpecifications=uint8(1)
  wires:
  Constant/1 -> ThdRwRtStFwdBkwdEn_Set/1

== system VIPRExit557StEnCtrl/VIPRExit557StEnCtrl_Cal_sys/If Action Subsystem19 ==
  Action Port : ActionPort  ActionType=else
  Constant : Constant  Value=27  OutDataTypeStr=uint8
  PassStFwdBkwdEn_Clear : FunctionCaller  FunctionPrototype=PassStFwdBkwdEn_Clear(data)  InputArgumentSpecifications=uint8(1)
  wires:
  Constant/1 -> PassStFwdBkwdEn_Clear/1

== system VIPRExit557StEnCtrl/VIPRExit557StEnCtrl_Cal_sys/If Action Subsystem2 ==
  Action Port : ActionPort  ActionType=then
  Constant : Constant  Value=27  OutDataTypeStr=uint8
  SecRwRtStFwdBkwdEn_Set : FunctionCaller  FunctionPrototype=SecRwRtStFwdBkwdEn_Set(data)  InputArgumentSpecifications=uint8(1)
  wires:
  Constant/1 -> SecRwRtStFwdBkwdEn_Set/1

== system VIPRExit557StEnCtrl/VIPRExit557StEnCtrl_Cal_sys/If Action Subsystem20 ==
  Action Port : ActionPort  ActionType=then
  Constant : Constant  Value=27  OutDataTypeStr=uint8
  PassStFwdBkwdEn_Set : FunctionCaller  FunctionPrototype=PassStFwdBkwdEn_Set(data)  InputArgumentSpecifications=uint8(1)
  wires:
  Constant/1 -> PassStFwdBkwdEn_Set/1

== system VIPRExit557StEnCtrl/VIPRExit557StEnCtrl_Cal_sys/If Action Subsystem21 ==
  Action Port : ActionPort  ActionType=else
  Constant : Constant  Value=27  OutDataTypeStr=uint8
  PassStBkReclnEn_Clear : FunctionCaller  FunctionPrototype=PassStBkReclnEn_Clear(data)  InputArgumentSpecifications=uint8(1)
  wires:
  Constant/1 -> PassStBkReclnEn_Clear/1

== system VIPRExit557StEnCtrl/VIPRExit557StEnCtrl_Cal_sys/If Action Subsystem22 ==
  Action Port : ActionPort  ActionType=then
  Constant : Constant  Value=27  OutDataTypeStr=uint8
  PassStBkReclnEn_Set : FunctionCaller  FunctionPrototype=PassStBkReclnEn_Set(data)  InputArgumentSpecifications=uint8(1)
  wires:
  Constant/1 -> PassStBkReclnEn_Set/1

== system VIPRExit557StEnCtrl/VIPRExit557StEnCtrl_Cal_sys/If Action Subsystem3 ==
  note: Delete block
  note: Delete block
  Action Port : ActionPort  ActionType=else
  Constant : Constant  Value=27  OutDataTypeStr=uint8
  ThdRwLtStBkReclnEn_Clear : FunctionCaller  FunctionPrototype=ThdRwLtStBkReclnEn_Clear(data)  InputArgumentSpecifications=uint8(1)
  wires:
  Constant/1 -> ThdRwLtStBkReclnEn_Clear/1

== system VIPRExit557StEnCtrl/VIPRExit557StEnCtrl_Cal_sys/If Action Subsystem4 ==
  note: Delete block
  note: Delete block
  Action Port : ActionPort  ActionType=then
  Constant : Constant  Value=27  OutDataTypeStr=uint8
  ThdRwLtStBkReclnEn_Set : FunctionCaller  FunctionPrototype=ThdRwLtStBkReclnEn_Set(data)  InputArgumentSpecifications=uint8(1)
  wires:
  Constant/1 -> ThdRwLtStBkReclnEn_Set/1

== system VIPRExit557StEnCtrl/VIPRExit557StEnCtrl_Cal_sys/If Action Subsystem5 ==
  note: Delete block
  note: Delete block
  Action Port : ActionPort  ActionType=else
  Constant : Constant  Value=27  OutDataTypeStr=uint8
  ThdRwLtStFwdBkwdEn_Clear : FunctionCaller  FunctionPrototype=ThdRwLtStFwdBkwdEn_Clear(data)  InputArgumentSpecifications=uint8(1)
  wires:
  Constant/1 -> ThdRwLtStFwdBkwdEn_Clear/1

== system VIPRExit557StEnCtrl/VIPRExit557StEnCtrl_Cal_sys/If Action Subsystem6 ==
  note: Delete block
  note: Delete block
  Action Port : ActionPort  ActionType=then
  Constant : Constant  Value=27  OutDataTypeStr=uint8
  ThdRwLtStFwdBkwdEn_Set : FunctionCaller  FunctionPrototype=ThdRwLtStFwdBkwdEn_Set(data)  InputArgumentSpecifications=uint8(1)
  wires:
  Constant/1 -> ThdRwLtStFwdBkwdEn_Set/1

== system VIPRExit557StEnCtrl/VIPRExit557StEnCtrl_Cal_sys/If Action Subsystem7 ==
  Action Port : ActionPort  ActionType=else
  Constant : Constant  Value=27  OutDataTypeStr=uint8
  SecRwRtStLgrstUpwdDnwdEn_Clear : FunctionCaller  FunctionPrototype=SecRwRtStLgrstUpwdDnwdEn_Clear(data)  InputArgumentSpecifications=uint8(1)
  wires:
  Constant/1 -> SecRwRtStLgrstUpwdDnwdEn_Clear/1

== system VIPRExit557StEnCtrl/VIPRExit557StEnCtrl_Cal_sys/If Action Subsystem8 ==
  Action Port : ActionPort  ActionType=then
  Constant : Constant  Value=27  OutDataTypeStr=uint8
  SecRwRtStLgrstUpwdDnwdEn_Set : FunctionCaller  FunctionPrototype=SecRwRtStLgrstUpwdDnwdEn_Set(data)  InputArgumentSpecifications=uint8(1)
  wires:
  Constant/1 -> SecRwRtStLgrstUpwdDnwdEn_Set/1

== system VIPRExit557StEnCtrl/VIPRExit557StEnCtrl_Cal_sys/If Action Subsystem9 ==
  Action Port : ActionPort  ActionType=else
  Constant : Constant  Value=27  OutDataTypeStr=uint8
  SecRwRtStLgrstInwdOtwdEn_Clear : FunctionCaller  FunctionPrototype=SecRwRtStLgrstInwdOtwdEn_Clear(data)  InputArgumentSpecifications=uint8(1)
  wires:
  Constant/1 -> SecRwRtStLgrstInwdOtwdEn_Clear/1

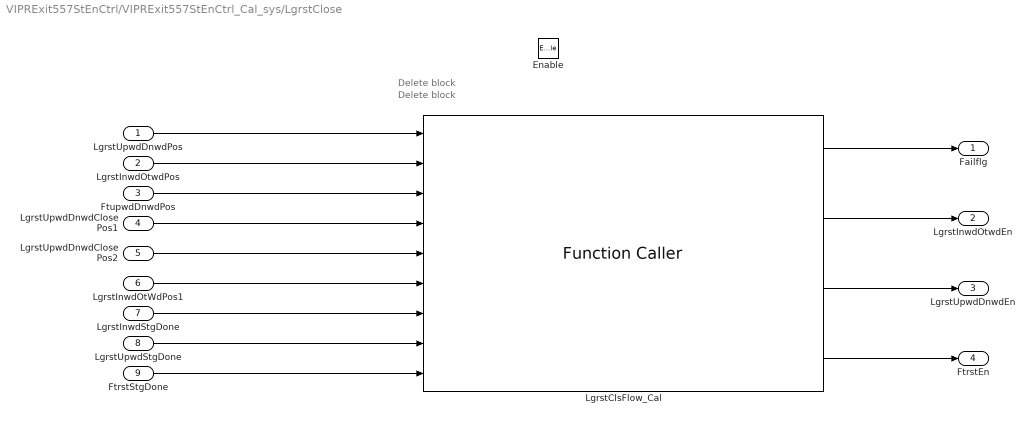
== system VIPRExit557StEnCtrl/VIPRExit557StEnCtrl_Cal_sys/LgrstClose ==
  note: Delete block
  note: Delete block
  LgrstUpwdDnwdPos : Inport
  LgrstInwdOtwdPos : Inport  Port=2
  FtupwdDnwdPos : Inport  Port=3
  LgrstUpwdDnwdClosePos1 : Inport  Port=4
  LgrstUpwdDnwdClosePos2 : Inport  Port=5
  LgrstInwdOtWdPos1 : Inport  Port=6
  LgrstInwdStgDone : Inport  Port=7
  LgrstUpwdStgDone : Inport  Port=8
  FtrstStgDone : Inport  Port=9
  Enable : EnablePort  StatesWhenEnabling=reset
  LgrstClsFlow_Cal : FunctionCaller  FunctionPrototype=[Failflg,LgrstInwdOtwdEn,LgrstUpwdDnwdEn,FtrstEn] = LgrstClsFlow_Cal(LgrstUpwdDnwdPos,LgrstOtwdInwdPos,FtUpwdDnwdPos,CloseDnwdPos1,CloseDnwdPos2,CloseOtwdPos1,LgrstInwdStgDone,LgrstUpwdStgDone,FtrstStgDone)  InputArgumentSpecifications=uint16(1), uint16(1), uint16(1), uint16(1), uint16(1), uint16(1), boolean(true), boolean(true), boolean(true)  OutputArgumentSpecifications=boolean(true), boolean(true), boolean(true), boolean(true)
  Failflg : Outport
  LgrstInwdOtwdEn : Outport  Port=2
  LgrstUpwdDnwdEn : Outport  Port=3
  FtrstEn : Outport  Port=4
  wires:
  LgrstClsFlow_Cal/1 -> Failflg/1
  LgrstClsFlow_Cal/4 -> FtrstEn/1
  LgrstClsFlow_Cal/3 -> LgrstUpwdDnwdEn/1
  LgrstUpwdDnwdPos/1 -> LgrstClsFlow_Cal/1
  LgrstClsFlow_Cal/2 -> LgrstInwdOtwdEn/1
  LgrstUpwdDnwdClosePos1/1 -> LgrstClsFlow_Cal/4
  LgrstUpwdStgDone/1 -> LgrstClsFlow_Cal/8
  LgrstInwdStgDone/1 -> LgrstClsFlow_Cal/7
  FtrstStgDone/1 -> LgrstClsFlow_Cal/9
  LgrstUpwdDnwdClosePos2/1 -> LgrstClsFlow_Cal/5
  LgrstInwdOtWdPos1/1 -> LgrstClsFlow_Cal/6
  LgrstInwdOtwdPos/1 -> LgrstClsFlow_Cal/2
  FtupwdDnwdPos/1 -> LgrstClsFlow_Cal/3

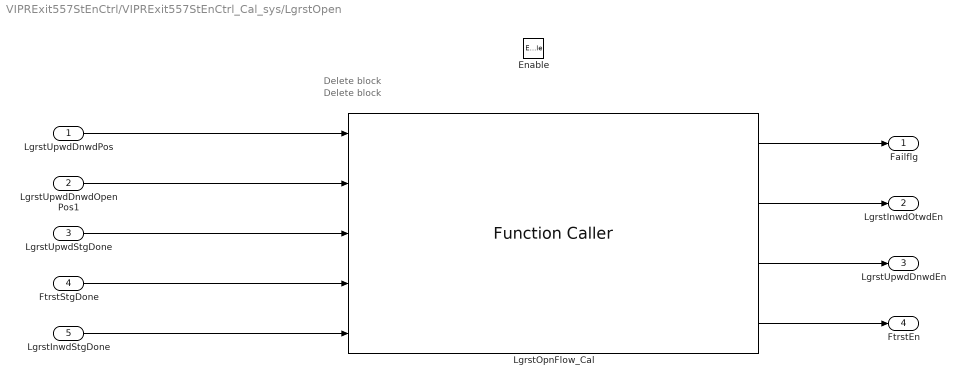
== system VIPRExit557StEnCtrl/VIPRExit557StEnCtrl_Cal_sys/LgrstOpen ==
  note: Delete block
  note: Delete block
  LgrstUpwdDnwdPos : Inport
  LgrstUpwdDnwdOpenPos1 : Inport  Port=2
  LgrstUpwdStgDone : Inport  Port=3
  FtrstStgDone : Inport  Port=4
  LgrstInwdStgDone : Inport  Port=5
  Enable : EnablePort  StatesWhenEnabling=reset
  LgrstOpnFlow_Cal : FunctionCaller  FunctionPrototype=[Failflg,LgrstInwdOtwdEn,LgrstUpwdDnwdEn,FtrstEn] = LgrstOpnFlow_Cal(LgrstUpwdDnwdPos,LgrstUpwdDnwdOpenPos1,LgrstUpwdStgDone,FtrstStgDone,LgrstInwdStgDone)  InputArgumentSpecifications=uint16(1), uint16(1), boolean(true), boolean(true), boolean(true)  OutputArgumentSpecifications=boolean(true), boolean(true), boolean(true), boolean(true)
  Failflg : Outport
  LgrstInwdOtwdEn : Outport  Port=2
  LgrstUpwdDnwdEn : Outport  Port=3
  FtrstEn : Outport  Port=4
  wires:
  LgrstOpnFlow_Cal/2 -> LgrstInwdOtwdEn/1
  LgrstUpwdDnwdPos/1 -> LgrstOpnFlow_Cal/1
  LgrstOpnFlow_Cal/3 -> LgrstUpwdDnwdEn/1
  FtrstStgDone/1 -> LgrstOpnFlow_Cal/4
  LgrstUpwdStgDone/1 -> LgrstOpnFlow_Cal/3
  LgrstOpnFlow_Cal/4 -> FtrstEn/1
  LgrstInwdStgDone/1 -> LgrstOpnFlow_Cal/5
  LgrstUpwdDnwdOpenPos1/1 -> LgrstOpnFlow_Cal/2
  LgrstOpnFlow_Cal/1 -> Failflg/1

== stateflow chart VIPRExit557StEnCtrl/VIPRExit557StEnCtrl_Cal_sys/Chart ==
  (default) -> (junction 228) : {
      | ThdRwLtStBkReclnEn = 0;
      | SecRwLtStBkReclnEn = 0;
      | SecRwLtStFrwdBkwdEn = 0;
      | SecRwLtStLgrstOtwdInwdEn = 0;
      | SecRwLtStLgrstUpwdDnwdEn = 0;
      | ThdRwLtStFwdBkwdEn = 0;
      | ZeroLEn = 0;
      | LgrstOpnEn = 0;
      | LgrstClsEn = 0;
      | PassStFwdBkwdEn = 0;
      | PassStBkReclnEn = 0;
      | ThdRwRtStBkReclnEn = 0;
      | ThdRwRtStFwdBkwdEn = 0;
      | }
  (junction 228) -> (junction 230) [order 1] : [(IfVeSMSuPassStBkReclnUpwdDnwdPos>VIPRExitPassStBkReclnUpwdDnwdTrgtPos)&&...
      | !NotMovPassStFlg&&!PassStBkReclnStgDone]
  (junction 228) -> (junction 234) [order 2]
  (junction 230) -> (junction 232) : {PassStBkReclnEn = 1;}
  (junction 232) -> (junction 234)
  (junction 234) -> (junction 38)
  (junction 38) -> (junction 40) [order 1] : [IfVeSMSuSecRwLtStBkReclnUpwdDnwdPos>VIPLR2LBkReclnUpwdDnwdTrgtPos&&!SecRwLtStBkReclnStgDone]
  (junction 38) -> (junction 44) [order 2]
  (junction 40) -> (junction 42) : {SecRwLtStBkReclnEn = 1;}
  (junction 42) -> (junction 44)
  (junction 44) -> (junction 56)
  (junction 56) -> (junction 58) [order 1] : [LgrstMoveDirection == 1&& !LgrstStgDone]
  (junction 56) -> (junction 62) [order 2]
  (junction 58) -> (junction 60) : {
      | LgrstClsEn = 1;
      | }
  (junction 60) -> (junction 62)
  (junction 62) -> (junction 111)
  (junction 111) -> (junction 113) [order 1] : [IfVeSMSuSecRwLtStZeroPos >VIPLMdR2LZeroTrgtPos && !ZeroLStgDone]
  (junction 111) -> (junction 117) [order 2]
  (junction 113) -> (junction 115) : {ZeroLEn = 1;}
  (junction 115) -> (junction 117)
  (junction 117) -> (junction 147)
  (junction 147) -> (junction 149) [order 1] : [!R3LMdSeatOccupied&&...
      | IfVeSMSuThdRwLtStBkReclnUpwdDnwdPos>VIPRExitR3LBkReclnUpwdDnwdTrgtPos&&...
      | !ThdRwLtStBkReclnStgDone&&...
      | Is7s]
  (junction 147) -> (junction 153) [order 2]
  (junction 149) -> (junction 151) : {
      | ThdRwLtStBkReclnEn = 1;
      | }
  (junction 151) -> (junction 153)
  (junction 153) -> (junction 263)
  (junction 263) -> (junction 266) [order 1] : [!R3RMdSeatOccupied&&...
      | IfVeSMSuThdRwRtStBkReclnUpwdDnwdPos>VIPRExitR3RBkReclnUpwdDnwdTrgtPos&&...
      | !ThdRwRtStBkReclnStgDone]
  (junction 263) -> (junction 270) [order 2]
  (junction 266) -> (junction 268) : {
      | ThdRwRtStBkReclnEn = 1;
      | }
  (junction 268) -> (junction 270)
  (junction 270) -> (junction 65)
  (junction 65) -> (junction 67) [order 1] : [
      | !(((IfVeSMSuPassStBkReclnUpwdDnwdPos<=VIPRExitPassStBkReclnUpwdDnwdTrgtPos)||...
      | NotMovPassStFlg||PassStBkReclnStgDone)&&...
      | (IfVeSMSuSecRwLtStBkReclnUpwdDnwdPos<=VIPLR2LBkReclnUpwdDnwdTrgtPos||SecRwLtStBkReclnStgDone)&&...
      | (IfVeSMSuSecRwLtStZeroPos <=VIPLMdR2LZeroTrgtPos ||ZeroLStgDone)&&...
      | (LgrstMoveDirection !=1||LgrstStgDone)&&...
      | (R3LMdSeatOccupied||IfVeSMSuThdRwLtStBkReclnUpwdDnwdPos<=VIPRExitR3LBkReclnUpwdDnwdTrgtPos||ThdRwLtStBkReclnStgDone||!Is7s)&&...
      | (R3RMdSeatOccupied||IfVeSMSuThdRwRtStBkReclnUpwdDnwdPos<=VIPRExitR3RBkReclnUpwdDnwdTrgtPos||ThdRwRtStBkReclnStgDone))
      | ]
  (junction 65) -> (junction 156) [order 2]
  (junction 67) -> (junction 175)
  (junction 156) -> (junction 158) [order 1] : [SecRwLtStFrwdBkwdStgDone]
  (junction 156) -> (junction 162) [order 2] : {SecRwLtStFrwdBkwdEn =1;}
  (junction 158) -> (junction 160)
  (junction 160) -> (junction 162)
  (junction 162) -> (junction 87)
  (junction 87) -> (junction 166) [order 1] : [ThdRwLtStFwdBkwdStgDone||!Is7s]
  (junction 87) -> (junction 170) [order 2] : {ThdRwLtStFwdBkwdEn = 1;}
  (junction 166) -> (junction 168)
  (junction 168) -> (junction 170)
  (junction 170) -> (junction 241)
  (junction 241) -> (junction 243) [order 1] : [ThdRwRtStFwdBkwdStgDone]
  (junction 241) -> (junction 247) [order 2] : {ThdRwRtStFwdBkwdEn = 1;}
  (junction 243) -> (junction 245)
  (junction 245) -> (junction 247)
  (junction 247) -> (junction 250)
  (junction 250) -> (junction 252) [order 1] : [NotMovPassStFlg ||PassStFwdBkwdStgDone]
  (junction 250) -> (junction 258) [order 2] : {PassStFwdBkwdEn = 1;}
  (junction 252) -> (junction 254)
  (junction 254) -> (junction 258)
  (junction 258) -> (junction 173)
  (junction 173) -> (junction 175) [order 1] : [!SecRwLtStFrwdBkwdStgDone||(!ThdRwLtStFwdBkwdStgDone&&Is7s)||...
      | !ThdRwRtStFwdBkwdStgDone||...
      | (!PassStFwdBkwdStgDone &&!NotMovPassStFlg)]
  (junction 173) -> (junction 179) [order 2]
  (junction 175) -> (junction 177)
  (junction 179) -> (junction 181) [order 1] : [ !ZeroLStgDone]
  (junction 179) -> (junction 185) [order 2]
  (junction 181) -> (junction 183) : {ZeroLEn = 1;}
  (junction 183) -> (junction 185)
  (junction 185) -> (junction 188)
  (junction 188) -> (junction 190) [order 1] : [!SecRwLtStBkReclnStgDone]
  (junction 188) -> (junction 194) [order 2]
  (junction 190) -> (junction 192) : {SecRwLtStBkReclnEn = 1;}
  (junction 192) -> (junction 194)
  (junction 194) -> (junction 273)
  (junction 273) -> (junction 275) [order 1] : [!NotMovPassStFlg&&!PassStBkReclnStgDone]
  (junction 273) -> (junction 279) [order 2]
  (junction 275) -> (junction 277) : {PassStBkReclnEn = 1;}
  (junction 277) -> (junction 279)
  (junction 279) -> (junction 282)
  (junction 282) -> (junction 285) [order 1] : [!ThdRwRtStBkReclnStgDone]
  (junction 282) -> (junction 289) [order 2]
  (junction 285) -> (junction 287) : {
      | ThdRwRtStBkReclnEn = 1;
      | }
  (junction 287) -> (junction 289)
  (junction 289) -> (junction 302)
  (junction 302) -> (junction 304) [order 1] : [ThdRwLtStBkReclnStgDone||!Is7s]
  (junction 302) -> (junction 308) [order 2] : {
      | ThdRwLtStBkReclnEn = 1;
      | }
  (junction 304) -> (junction 306)
  (junction 306) -> (junction 308)
  (junction 308) -> (junction 197)
  (junction 197) -> (junction 199) [order 1] : [!LgrstStgDone]
  (junction 197) -> (junction 204) [order 2]
  (junction 199) -> (junction 201) : {LgrstOpnEn = 1;}
  (junction 201) -> (junction 204)
  (junction 177) -> (junction 201)
  (junction 204) -> (junction 261)
  data: IfVeSMSuSecRwLtStBkReclnUpwdDnwdPos input; IfVeSMSuSecRwLtStLgrstOtwdInwdPos input; IfVeSMSuSecRwLtStLgrstUpwdDnwdPos input; SecRwLtStBkReclnStgDone input; SecRwLtStFrwdBkwdStgDone input; SecRwLtStLgrstOtwdInwdStgDone input; SecRwLtStLgrstUpwdDnwdStgDone input; ThdRwLtStBkReclnStgDone input; ThdRwLtStFwdBkwdStgDone input; VIPLR2LBkReclnUpwdDnwdTrgtPos input; VIPLR2LLgrstInwdOtwdTrgtPos input; VIPLR2LLgrstUpwdDnwdTrgtPos input; SecRwLtStBkReclnEn output boolean; SecRwLtStFrwdBkwdEn output boolean; SecRwLtStLgrstOtwdInwdEn output boolean; ThdRwLtStBkReclnEn output boolean; ThdRwLtStFwdBkwdEn output boolean; SecRwLtStLgrstUpwdDnwdEn output boolean; ZeroLStgDone input; ZeroLEn output boolean; IfVeSMSuSecRwLtStZeroPos input; VIPLMdR2LZeroTrgtPos input; R3LMdSeatOccupied input; LgrstStgDone input; IfVeSMSuThdRwLtStBkReclnUpwdDnwdPos input; LgrstMoveDirection input uint8 =0; LgrstClsEn output boolean; LgrstOpnEn output boolean; IfVeSMSuThdRwRtStBkReclnUpwdDnwdPos input; NotMovPassStFlg input; R3RMdSeatOccupied input; StNumFlg_Is7s input; PassStBkReclnStgDone input; PassStFwdBkwdStgDone input; ThdRwRtStBkReclnStgDone input; ThdRwRtStFwdBkwdStgDone input; VIPRExitR3LBkReclnUpwdDnwdTrgtPos input; VIPRExitR3RBkReclnUpwdDnwdTrgtPos input; ThdRwRtStBkReclnEn output boolean; ThdRwRtStFwdBkwdEn output boolean; PassStFwdBkwdEn output boolean; PassStBkReclnEn output boolean; VIPRExitPassStBkReclnUpwdDnwdTrgtPos input; IfVeSMSuPassStBkReclnUpwdDnwdPos input; Is7s input
